simulink model "exp4"  (R2022b)
settings: Solver=VariableStepAuto  StartTime=0.0  StopTime=5  RelTol=1e-3
settings Model: Creator=IITP  LastModifiedBy=IITP

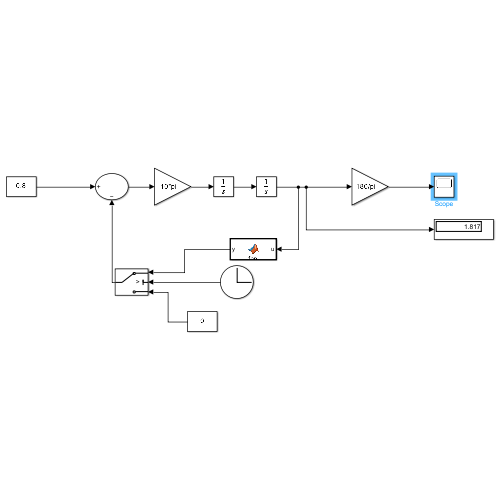
[thumbnail: Simulink's stored preview of the top-level diagram]
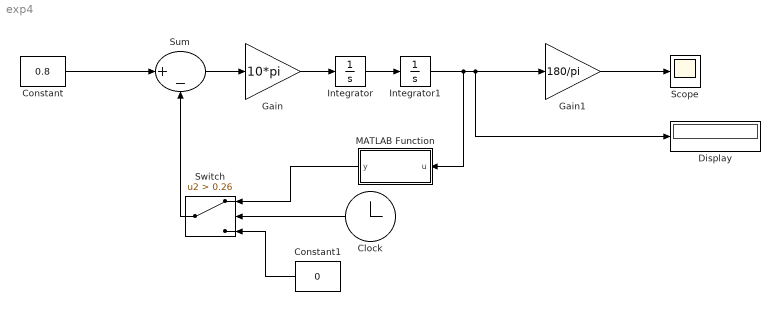
== system exp4 ==
  Clock : Clock
  Constant : Constant  Value=0.8
  Constant1 : Constant  Value=0
  Display : Display
  Gain : Gain  Gain=10*pi
  Gain1 : Gain  Gain=180/pi
  Integrator : Integrator
  Integrator1 : Integrator  InitialCondition=0.46
  MATLAB Function : MATLAB Function  TreatAsAtomicUnit=on
  Scope : Scope
  Sum : Sum  Inputs=|+-
  Switch : Switch  Criteria=u2 > Threshold  Threshold=0.26  SaturateOnIntegerOverflow=off  InputSameDT=off
  wires:
  Constant/1 -> Sum/1
  Sum/1 -> Gain/1
  Gain/1 -> Integrator/1
  Clock/1 -> Switch/2
  Switch/1 -> Sum/2
  Integrator/1 -> Integrator1/1
  Integrator1/1 -> MATLAB Function/1(u), Display/1, Gain1/1
  MATLAB Function/1(y) -> Switch/1
  Constant1/1 -> Switch/3
  Gain1/1 -> Scope/1

== matlab function exp4/MATLAB Function ==
  data: u input; y output
function y = fcn(u)

y = 1.8*sin(u);
